simulink model "OptimalControl"  (R2022b)
settings: Solver=ode45  StartTime=0.0  StopTime=pi  RelTol=1e-3
InitFcn:
  | A_sys = [-1,1;1,0];
  | B_sys = [2;1];
  | 
  | K = [0.9821,1.6726];
  | r = 2;
  | Q = [3,0;0,5];
settings Model: Creator=zein  LastModifiedBy=zein

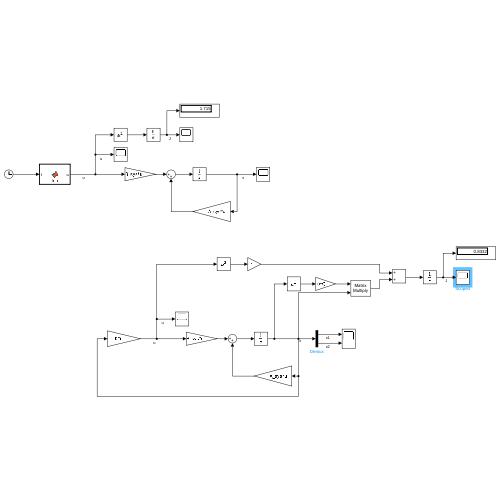
[thumbnail: Simulink's stored preview of the top-level diagram]
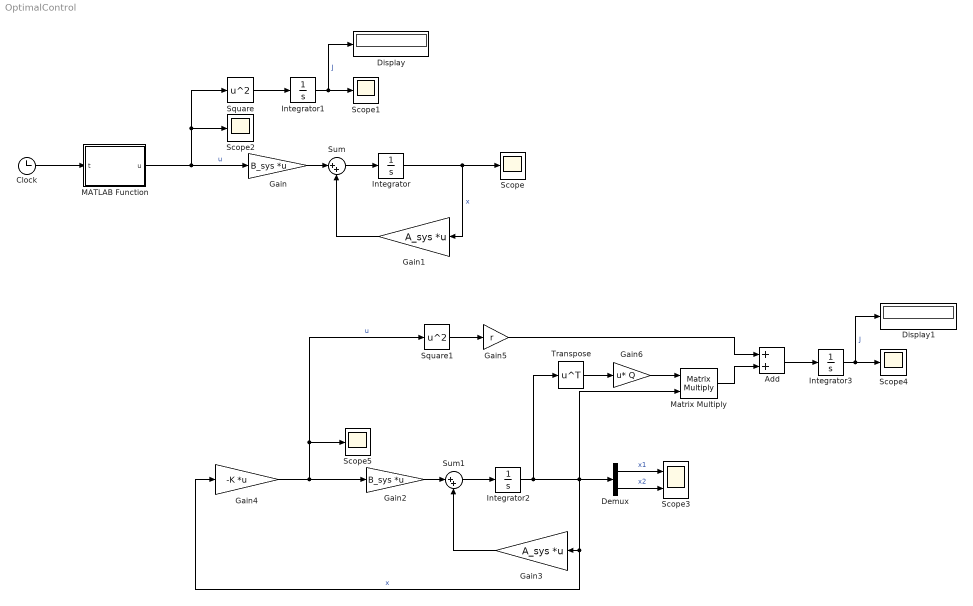
== system OptimalControl ==
  Add : Sum
  Clock : Clock
  Demux : Demux  Outputs=2
  Display : Display
  Display1 : Display
  Gain : Gain  Gain=B_sys  Multiplication=Matrix(K*u)
  Gain1 : Gain  Gain=A_sys  Multiplication=Matrix(K*u)
  Gain2 : Gain  Gain=B_sys  Multiplication=Matrix(K*u)
  Gain3 : Gain  Gain=A_sys  Multiplication=Matrix(K*u)
  Gain4 : Gain  Gain=-K  Multiplication=Matrix(K*u)
  Gain5 : Gain  Gain=r
  Gain6 : Gain  Gain=Q  Multiplication=Matrix(u*K)
  Integrator : Integrator  InitialCondition=[-0.9243;0]
  Integrator1 : Integrator
  Integrator2 : Integrator  InitialCondition=[1;0]
  Integrator3 : Integrator
  MATLAB Function : MATLAB Function  TreatAsAtomicUnit=on
  Matrix Multiply : Product  Multiplication=Matrix(*)
  Scope{,1..2,4..5} (5 alike) : Scope
  Scope3 : Scope  NumInputPorts=2
  Square : Math  Operator=square
  Square1 : Math  Operator=square
  Sum : Sum  Inputs=|++
  Sum1 : Sum  Inputs=|++
  Transpose : Math  Operator=transpose
  wires:
  Clock/1 -> MATLAB Function/1(t)
  Gain/1 -> Sum/1
  Sum/1 -> Integrator/1
  MATLAB Function/1(u) -> Square/1, Scope2/1, Gain/1  "u"
  Integrator/1 -> Scope/1, Gain1/1  "x"
  Gain1/1 -> Sum/2
  Square/1 -> Integrator1/1
  Integrator1/1 -> Display/1, Scope1/1  "J"
  Integrator2/1 -> Transpose/1, Gain3/1, Gain4/1, Demux/1, Matrix Multiply/2  "x"
  Gain4/1 -> Scope5/1, Square1/1, Gain2/1  "u"
  Integrator3/1 -> Display1/1, Scope4/1  "J"
  Gain3/1 -> Sum1/2
  Sum1/1 -> Integrator2/1
  Square1/1 -> Gain5/1
  Gain2/1 -> Sum1/1
  Gain5/1 -> Add/1
  Add/1 -> Integrator3/1
  Matrix Multiply/1 -> Add/2
  Transpose/1 -> Gain6/1
  Gain6/1 -> Matrix Multiply/1
  Demux/1 -> Scope3/1  "x1"
  Demux/2 -> Scope3/2  "x2"

== matlab function OptimalControl/MATLAB Function ==
  data: t input; u output
function u = fcn(t)
u = (exp(t./2.0+pi).*(exp((pi.*(sqrt(5.0).*3.0-1.0))./2.0)-exp(pi.*(-1.0./2.0)+(sqrt(5.0).*pi)./2.0+sqrt(5.0).*t)+exp(pi.*(-1.0./2.0)+sqrt(5.0).*pi.*(3.0./2.0)+sqrt(5.0).*t)-exp((pi.*(sqrt(5.0)-1.0))./2.0)+sqrt(5.0).*exp(pi.*(-1.0./2.0)+(sqrt(5.0).*pi)./2.0+sqrt(5.0).*t)-sqrt(5.0).*exp(pi.*(-1.0./2.0)+sqrt(5.0).*pi.*(3.0./2.0)+sqrt(5.0).*t)-sqrt(5.0).*exp((pi.*(sqrt(5.0)-1.0))./2.0)+sqrt(5.0).*exp((pi.*(sqrt(5.0).*3.0-1.0))./2.0)))./(exp(pi+(sqrt(5.0).*t)./2.0).*5.0-exp(pi+sqrt(5.0).*pi.*2.0+(sqrt(5.0).*t)./2.0).*5.0+sqrt(5.0).*exp(pi+(sqrt(5.0).*t)./2.0).*2.0+sqrt(5.0).*exp(pi+sqrt(5.0).*pi+(sqrt(5.0).*t)./2.0).*4.0+sqrt(5.0).*exp(pi+sqrt(5.0).*pi.*2.0+(sqrt(5.0).*t)./2.0).*2.0-sqrt(5.0).*exp(sqrt(5.0).*(t./2.0+pi)).*8.0);
